simulink model "longmendiao_SA"  (R2022b)
settings: Solver=VariableStepAuto  StartTime=0.0  StopTime=20  RelTol=1e-3
settings Model: Creator=MasterMo  LastModifiedBy=47800
settings SolverCC: AlgebraicLoopSolver=TrustRegion
settings DebuggingCC: UnconnectedInputMsg=warning  UnconnectedOutputMsg=warning  UnconnectedLineMsg=warning  SFMachineParentedDataDiag=warning  ArithmeticOperatorsInVariantConditions=warning
settings ModelReferenceCC: EnableRefExpFcnMdlSchedulingChecks=on
settings SFSimCC: CustomCodeUndefinedFunction=UseInterfaceOnly
settings CodeAppCC: StateflowObjectComments=on

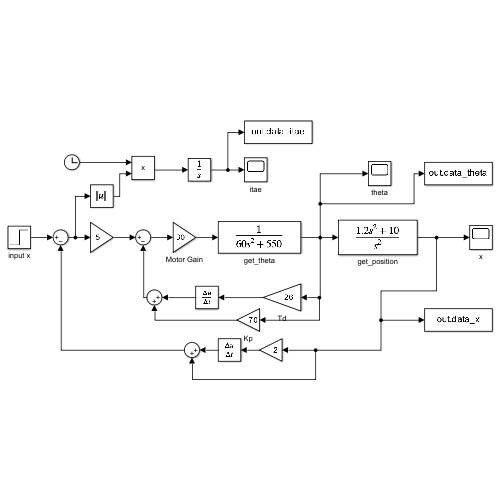
[thumbnail: Simulink's stored preview of the top-level diagram]
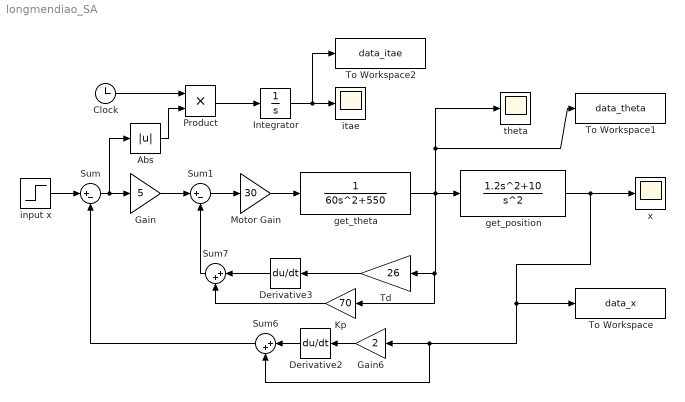
== system longmendiao_SA ==
  Abs : Abs  SaturateOnIntegerOverflow=off
  Clock : Clock
  Derivative2 : Derivative
  Derivative3 : Derivative
  Gain : Gain  Gain=5
  Gain6 : Gain  Gain=2
  Integrator : Integrator
  Kp : Gain  Gain=70
  Motor Gain : Gain  Gain=30
  Product : Product
  Sum : Sum  Inputs=|+-
  Sum1 : Sum  Inputs=|+-
  Sum6 : Sum  Inputs=|++
  Sum7 : Sum  Inputs=|++
  Td : Gain  Gain=26
  To Workspace : ToWorkspace  VariableName=data_x  SaveFormat=Structure With Time  SampleTime=-1
  To Workspace1 : ToWorkspace  VariableName=data_theta  SaveFormat=Structure With Time  SampleTime=-1
  To Workspace2 : ToWorkspace  VariableName=data_itae  SaveFormat=Structure With Time  SampleTime=-1
  get_position : TransferFcn  Numerator=[1.2 0 10]  Denominator=[1 0 0]
  get_theta : TransferFcn  Denominator=[60 0 550]
  input x : Step  After=8  SampleTime=0
  "itae " : Scope
  theta : Scope
  x : Scope
  wires:
  input x/1 -> Sum/1
  Motor Gain/1 -> get_theta/1
  Sum1/1 -> Motor Gain/1
  Gain/1 -> Sum1/1
  Sum/1 -> Abs/1, Gain/1
  Derivative2/1 -> Sum6/1
  Gain6/1 -> Derivative2/1
  get_position/1 -> Sum6/2, Gain6/1, To Workspace/1, x/1
  Sum6/1 -> Sum/2
  Td/1 -> Derivative3/1
  Sum7/1 -> Sum1/2
  Kp/1 -> Sum7/2
  Derivative3/1 -> Sum7/1
  get_theta/1 -> Kp/1, Td/1, To Workspace1/1, theta/1, get_position/1
  Clock/1 -> Product/1
  Product/1 -> Integrator/1
  Abs/1 -> Product/2
  Integrator/1 -> To Workspace2/1, "itae "/1
